simulink model "kite"  (Simulink 7.7)
settings: Solver=FixedStepDiscrete  StartTime=0.0  StopTime=T  FixedStep=Ts  RelTol=1e-3
InitFcn:
  | initialize
values from neighbouring files (symbols this model uses):
  state = TX(1,2:end)    [kiteData.m]
  Ts = 0.1    [initialize.m]
settings Model: Creator=pgoulart  LastModifiedBy=rien
settings DataIOCC: SaveOutput=off  DSMLogging=off  SaveTime=off  SignalLoggingName=craneLogger
settings DebuggingCC: UnderspecifiedInitializationDetection=Simplified  SolverPrmCheckMsg=none

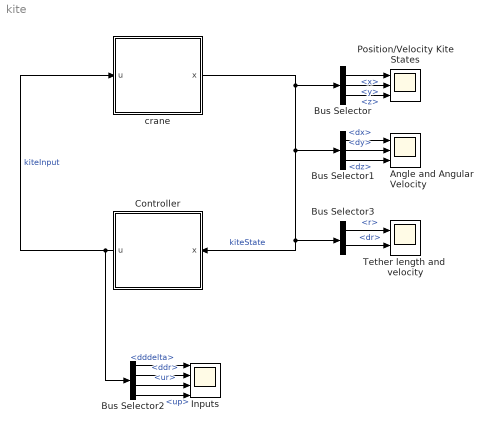
== system kite ==
  Angle and Angular Velocity : Scope  NumInputPorts=3
      settings: TimeRange=5  YMin=-5~-5~-5  YMax=5~5~5  SaveName=ScopeData2
  Bus Selector : BusSelector  OutputSignals=x,y,z
  Bus Selector1 : BusSelector  OutputSignals=dx,dy,dz
  Bus Selector2 : BusSelector  OutputSignals=dddelta,ddr,ur,up
  Bus Selector3 : BusSelector  OutputSignals=r,dr
  Controller : Subsystem
      mask Display: disp('Controller');
  Inputs : Scope  NumInputPorts=4
      settings: TimeRange=5  YMin=-4~-30~-10~-125  YMax=10~100~1~25
  Position/Velocity Kite States : Scope  NumInputPorts=3
      settings: TimeRange=5  YMin=-5~-5~-5  YMax=5~5~5
  Tether length and  velocity : Scope  NumInputPorts=2
      settings: TimeRange=5  YMin=-5~-5  YMax=5~5  SaveName=ScopeData3
  crane : Subsystem
      mask help: KU Leuven Kite Model. Edit <kiteData.m> for configuration.
      mask init:
      | % initialize state values
      | kiteData
      mask Display: disp('Kite');
  wires:
  Controller/1(u) -> crane/1(u), Bus Selector2/1  "kiteInput"
  crane/1(x) -> Bus Selector/1, Bus Selector1/1, Controller/1(x), Bus Selector3/1  "kiteState"
  Bus Selector/1 -> Position/Velocity Kite States/1  "<x>"
  Bus Selector/2 -> Position/Velocity Kite States/2  "<y>"
  Bus Selector/3 -> Position/Velocity Kite States/3  "<z>"
  Bus Selector1/1 -> Angle and Angular Velocity/1  "<dx>"
  Bus Selector1/2 -> Angle and Angular Velocity/2  "<dy>"
  Bus Selector2/1 -> Inputs/1  "<dddelta>"
  Bus Selector2/2 -> Inputs/2  "<ddr>"
  Bus Selector2/3 -> Inputs/3  "<ur>"
  Bus Selector2/4 -> Inputs/4  "<up>"
  Bus Selector1/3 -> Angle and Angular Velocity/3  "<dz>"
  Bus Selector3/1 -> Tether length and  velocity/1  "<r>"
  Bus Selector3/2 -> Tether length and  velocity/2  "<dr>"

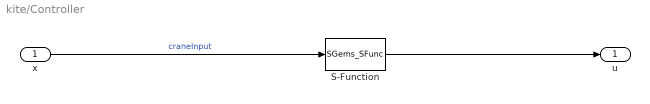
== system kite/Controller ==
  x : Inport
  S-Function : S-Function  FunctionName=SGems_SFunc  EnableBusSupport=off
  u : Outport
  wires:
  S-Function/1 -> u/1
  x/1 -> S-Function/1  "craneInput"

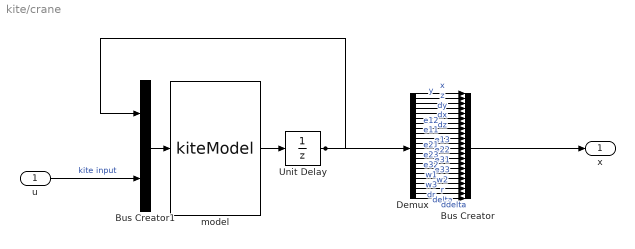
== system kite/crane ==
  u : Inport
  Bus Creator : BusCreator  Inputs='x','y','z','dx','dy','dz','e11','e12','e13','e21','e22','e23','e31','e32','e33','w1','w2','w3','r','dr','delta','ddelta'
  Bus Creator1 : BusCreator  Inputs=2
  Demux : Demux  Outputs=22
  Unit Delay : UnitDelay  X0=state  SampleTime=Ts
  model : S-Function  FunctionName=kiteModel  EnableBusSupport=off
  x : Outport
  wires:
  u/1 -> Bus Creator1/2  "kite input"
  Bus Creator1/1 -> model/1
  Demux/1 -> Bus Creator/1  "x"
  Demux/2 -> Bus Creator/2  "y"
  Demux/3 -> Bus Creator/3  "z"
  Demux/4 -> Bus Creator/4  "dx"
  Demux/5 -> Bus Creator/5  "dy"
  Demux/6 -> Bus Creator/6  "dz"
  Demux/7 -> Bus Creator/7  "e11"
  Demux/8 -> Bus Creator/8  "e12"
  Demux/9 -> Bus Creator/9  "e13"
  Demux/10 -> Bus Creator/10  "e21"
  Demux/11 -> Bus Creator/11  "e22"
  Demux/12 -> Bus Creator/12  "e23"
  Demux/13 -> Bus Creator/13  "e31"
  Demux/14 -> Bus Creator/14  "e32"
  Demux/15 -> Bus Creator/15  "e33"
  Demux/16 -> Bus Creator/16  "w1"
  Demux/17 -> Bus Creator/17  "w2"
  Demux/18 -> Bus Creator/18  "w3"
  Demux/19 -> Bus Creator/19  "r"
  Demux/20 -> Bus Creator/20  "dr"
  Demux/21 -> Bus Creator/21  "delta"
  Demux/22 -> Bus Creator/22  "ddelta"
  model/1 -> Unit Delay/1
  Unit Delay/1 -> Bus Creator1/1, Demux/1
  Bus Creator/1 -> x/1
